simulink model "MPC_pos"  (R2018b)
settings: Solver=VariableStepAuto  StartTime=0.0  StopTime=5  RelTol=1e-3
libraries: mpclib x1
settings Model: Creator=dongdaming  LastModifiedBy=dongdaming

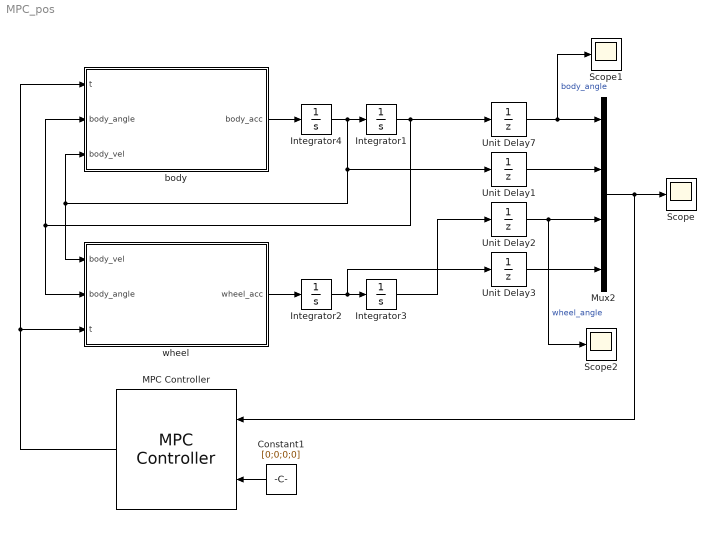
== system MPC_pos ==
  Constant1 : Constant  Value=[0;0;0;0]
  Integrator1 : Integrator  InitialCondition=1
  Integrator2 : Integrator
  Integrator3 : Integrator
  Integrator4 : Integrator
  MPC Controller : mpclib/MPC Controller  SCDEnableBlockLinearizationSpecification=on  mpcobj=mpc1  is_multiple=0  enable_value=0  return_u0=off  updateMPCinCallerWorkspace=on  md_inport=off  mv_inport=off  return_cost=off  return_mvseq=off  return_qpstatus=off  return_xseq=off  return_state=off  return_ovseq=off  state_inport=off  umin_inport=off  umax_inport=off  ymin_inport=off  ymax_inport=off  cc_inport=off  ywt_inport=off  uwt_inport=off  duwt_inport=off  rhoeps_inport=off  uref_inport=off  n_ts=0.002  n_p=10  n_mv=1  n_md=0  n_ud=0  n_mo=4  n_uo=0  BlockDataType=double  SampleTimeInherited=off  switch_inport=off
  Mux2 : Mux
  Scope : Scope
  Scope1 : Scope
  Scope2 : Scope
  Unit Delay{1..3,7} (4 alike) : UnitDelay  SampleTime=0.002
  body : MATLAB Function  TreatAsAtomicUnit=on
  wheel : MATLAB Function  TreatAsAtomicUnit=on
  wires:
  body/1(body_acc) -> Integrator4/1
  Integrator2/1 -> Unit Delay3/1, Integrator3/1
  Integrator4/1 -> wheel/1(body_vel), body/3(body_vel), Unit Delay1/1, Integrator1/1
  Integrator1/1 -> Unit Delay7/1, body/2(body_angle), wheel/2(body_angle)
  Unit Delay1/1 -> Mux2/2
  Unit Delay7/1 -> Scope1/1, Mux2/1  "body_angle"
  Mux2/1 -> MPC Controller/1, Scope/1
  Constant1/1 -> MPC Controller/2
  MPC Controller/1 -> body/1(t), wheel/3(t)
  Unit Delay2/1 -> Scope2/1, Mux2/3  "wheel_angle"
  Unit Delay3/1 -> Mux2/4
  Integrator3/1 -> Unit Delay2/1
  wheel/1(wheel_acc) -> Integrator2/1

== matlab function MPC_pos/wheel ==
  data: body_vel input; body_angle input; t input; wheel_acc output
function wheel_acc = wheel_model(body_vel,body_angle,t)
wheel_acc=(-1225.31*sin(2*body_angle)+(5377.69+2083.85*cos(body_angle))*t+20.005*sin(body_angle)*body_vel*body_vel)/(2.1931+cos(body_angle)*cos(body_angle)+8.75194*sin(body_angle)*sin(body_angle));

== matlab function MPC_pos/body ==
  data: t input; body_acc output; body_angle input; body_vel input
function body_acc = body_model(t,body_angle,body_vel)
body_acc=(+1429.48*sin(body_angle)-1215.55*t-2083.85*t*cos(body_angle)-3.87597*sin(2*body_angle)*body_vel^2)/(2.91931+cos(body_angle)^2+8.75194*sin(body_angle)^2);
